simulink model "board_unspecific_DataloggerSerial"  (R2015a)
settings: Solver=FixedStepDiscrete  SolverMode=SingleTasking  StartTime=0.0  StopTime=10.0  FixedStep=1e-3  RelTol=1e-3
libraries: mbed_lib x5, simulink x1
settings Model: Creator=oh  LastModifiedBy=oh
settings OptimizationCC: OptimizeModelRefInitCode=on  LifeSpan=1
settings HardwareCC: ProdLargestAtomicInteger=Long  ProdLargestAtomicFloat=Double  ProdEndianess=LittleEndian  ProdHWDeviceType=ARM Compatible->ARM Cortex
settings RTWCC: SystemTargetFile=mbed.tlc  TemplateMakefile=mbed.tmf  Description=Mbed Target (Embedded Target)  TargetLang=C++
settings CodeAppCC: IgnoreCustomStorageClasses=off
settings STFCustomTargetCC: CombineOutputUpdateFcns=on  SupportContinuousTime=off  SupportVariableSizeSignals=off  SystemTargetFile=mbed.tlc
settings ERTTargetCC: SupportContinuousTime=off  SupportVariableSizeSignals=off  ERTCustomFileTemplate=mbed_file_process.tlc

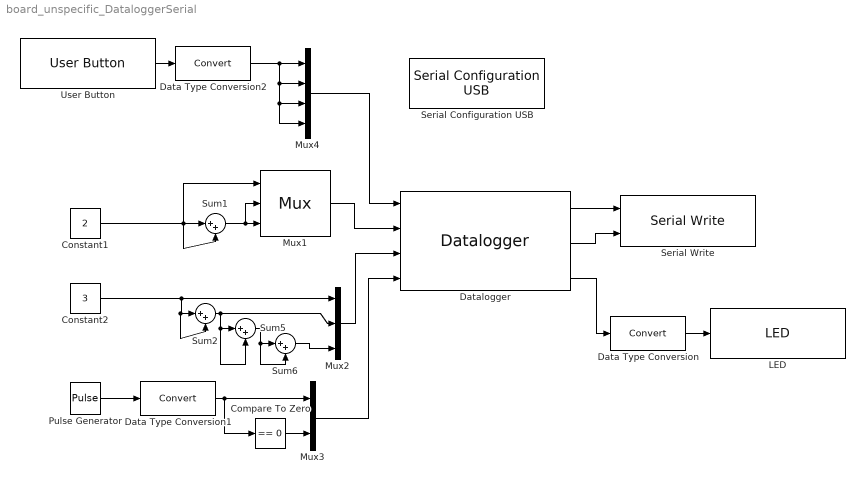
== system board_unspecific_DataloggerSerial ==
  Compare To Zero : simulink/Logic and Bit Operations/Compare To Zero  relop===  OutDataTypeStr=boolean
  Constant1 : Constant  Value=2  OutDataTypeStr=int16
  Constant2 : Constant  Value=3
  Data Type Conversion1 : DataTypeConversion
  Data Type Conversion2 : DataTypeConversion
  Data Type Conversion : DataTypeConversion
  Datalogger : mbed_lib/Utilities/Datalogger  TypeInputPorts={ 'uint8' 4 'int16' 3 'double' 3 'bool' 2 }  TypeOfInputs={'4*uint8' '3*int16' '3*double' '2*bool'}  BufferSize=120  errEn=on  SampleTime=1
  LED : mbed_lib/GPIO/LED  nLED=1  SampleTime=-1
  Mux1 : Mux  Inputs=3
      settings: DisplayOption=signals
  Mux2 : Mux  Inputs=3
  Mux3 : Mux  Inputs=2
  Mux4 : Mux
  Pulse Generator : DiscretePulseGenerator  PulseType=Time based  Period=1  PulseWidth=50
  Serial Configuration USB : mbed_lib/Serial/UART/Serial Configuration USB  BaudRate=9600
  Serial Write : mbed_lib/Serial/UART/Serial Write  SerialPort=0  numData=on  SampleTime=-1
  Sum{1..2,5..6} (4 alike) : Sum  Inputs=|++
  User Button : mbed_lib/GPIO/User Button  SampleTime=-1
  wires:
  Sum1/1 -> Mux1/2, Mux1/3
  Sum2/1 -> Mux2/2, Sum5/2, Sum5/1
  Constant1/1 -> Mux1/1, Sum1/2, Sum1/1
  Constant2/1 -> Mux2/1, Sum2/2, Sum2/1
  Sum5/1 -> Sum6/2, Sum6/1
  Pulse Generator/1 -> Data Type Conversion1/1
  Sum6/1 -> Mux2/3
  Mux2/1 -> Datalogger/3
  Mux1/1 -> Datalogger/2
  Mux3/1 -> Datalogger/4
  User Button/1 -> Data Type Conversion2/1
  Mux4/1 -> Datalogger/1
  Compare To Zero/1 -> Mux3/2
  Datalogger/1 -> Serial Write/1
  Datalogger/2 -> Serial Write/2
  Datalogger/3 -> Data Type Conversion/1
  Data Type Conversion/1 -> LED/1
  Data Type Conversion1/1 -> Compare To Zero/1, Mux3/1
  Data Type Conversion2/1 -> Mux4/4, Mux4/3, Mux4/2, Mux4/1
